simulink model "ShapeTracingSimExample"  (R2025b)
settings: Solver=VariableStepAuto  StartTime=0.0  StopTime=inf  RelTol=1e-3
InitFcn:
  | robotMesh = importrobot('ur5e_with_gripper.urdf');
undefined symbols (not defined in the file or in its folder): Sim3dSensor
libraries: sim3dlib x3, shareduavrstlib x1, sim3dphyssensorlib x1, robotsim3dlib x1, simulink x1, visionsinks x1
settings Model: Creator=The MathWorks, Inc.  LastModifiedBy=pepadev

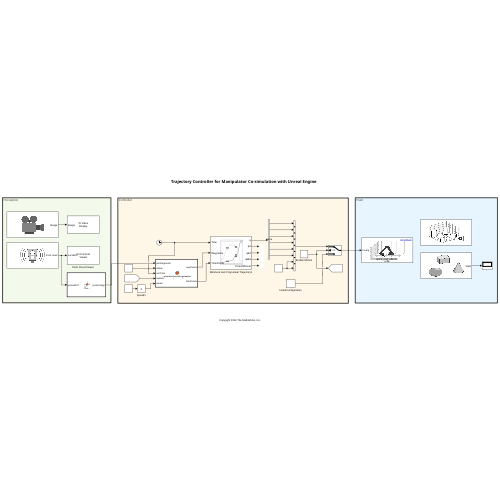
[thumbnail: Simulink's stored preview of the top-level diagram]
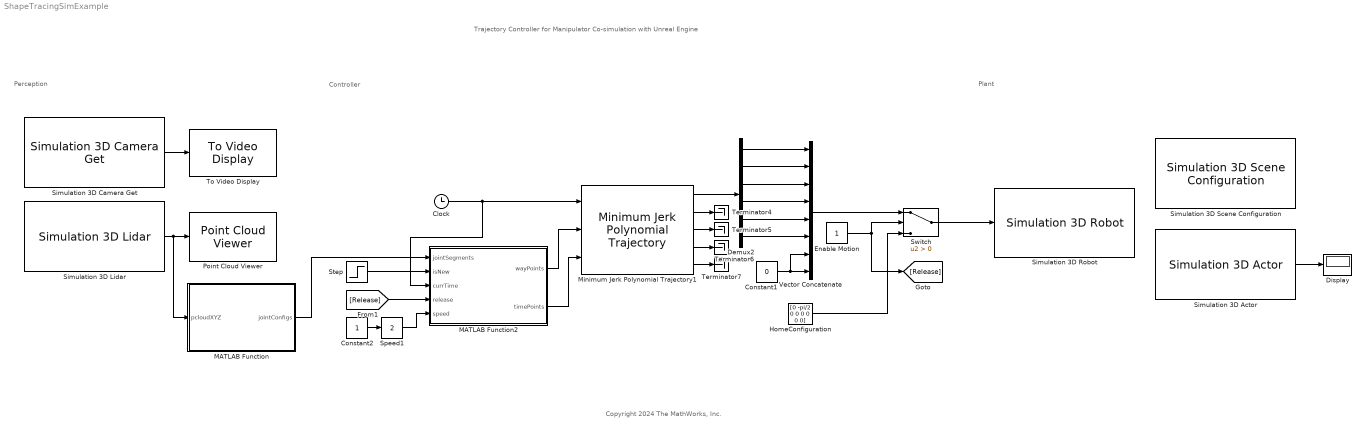
== system ShapeTracingSimExample ==
  note: Trajectory Controller for Manipulator Co-simulation with Unreal Engine
  note: Copyright 2024 The MathWorks, Inc.
  note: Plant
  note: Controller
  note: Perception
  Clock : Clock
  Constant1 : Constant  Value=0
  Constant2 : Constant
  Demux2 : Demux  Outputs=6
      settings: DisplayOption=none
  Display : Display
  Enable Motion : Constant
  HomeConfiguration : Constant  Value=|
      | [0
      | -pi/2
      | 0
      | 0
      | 0
      | 0
      | 0
      | 0]
  MATLAB Function : MATLAB Function  TreatAsAtomicUnit=on
  MATLAB Function2 : MATLAB Function  TreatAsAtomicUnit=on
  Minimum Jerk Polynomial Trajectory1 : shareduavrstlib/Minimum Jerk Polynomial Trajectory  ShowBCInputPort=off  ShowPolynomialCoefs=off  ShowStatusOutputPort=off  TimeAllocation=off  TimeWeight=100  MinSegmentTime=0.1  MaxSegmentTime=1  MaxIteration=1500  MaxTime=10  SimulateUsing=Interpreted execution
      settings: LibrarySourceBlock=robotutilslib/Minimum Jerk Polynomial Trajectory
  Point Cloud Viewer : PointCloudViewer  FigPos=[15.6666666666667 748.666666666667 1264 670.666666666667]  OpenAtMdlStart=off
  Simulation 3D Actor : sim3dlib/Simulation 3D Actor  Priority=1  ActorName=Actor1  ParentName=Scene Origin  Operation=Create at setup  InitScriptText=|  SampleTime=-1  Translation=single([0 0 0])  Rotation=single([0 0 0])  Scale=single([1 1 1])  aMode=5  ActorTag=Actor1  ActorType=Sim3dActor  ID=C
      | % Reserved keywords:
      | % - Actor : handle to this actor object
      | % - World : handle to the world object
      | 
      | % Examples:
      | 
      | % Create a primitive geometry (optional)
      | % Actor.createShape('box', [1 1 1]);
      | 
      | % Initialize values (optional)
      | % Actor.Scale = 1;
      | % Actor.Color = [1 0 0];
  Simulation 3D Camera Get : sim3dlib/Simulation 3D Camera Get  Priority=1  sensorTag=Sim3dSensor�  sensorId=1  sensorName=Sim3dSensor�  vehTagList={'Actor1';'Scene Origin';'ur5e'}  vehTag=ur5e  CoordinateSystem=Default  mountLoc=Origin  offsetFlag=on  tmountOffset=[- 5 0 3]  rmountOffset=[0 30 0]  HorizontalResolution=1280  VerticalResolution=720  HorizontalFOV=60  SampleTime=-1  mountPoint=[-5 0 3]  mountOrientation=[0 30 0]  aMode=5  ID=1
      settings: LibrarySourceBlock=sl3dlib/Simulation 3D/Utilities/Simulation 3D Camera Get
  Simulation 3D Lidar : sim3dphyssensorlib/Simulation 3D Lidar  Priority=1  sensorTag=Sim3dSensor�  sensorId=2  sensorName=Sim3dSensor�  vehTagList={'Actor1';'Scene Origin';'ur5e'}  vehTag=ur5e  CoordinateSystem=Default  mountLoc=Origin  offsetFlag=on  tmountOffset=[0, 0.25, 0.1]  rmountOffset=[0, 0, 90]  DetectionRange=1  RangeResolution=0.0001  VerticalFOV=48  VerticalResolution=0.1  HorizontalFOV=128  HorizontalResolution=0.2  DistanceOutportEnabled=off  ReflectivityOutportEnabled=off  SemanticOutportEnabled=off  TransformOutportEnabled=off  SampleTime=-1  mountPoint=[0 0.25 0.1]  mountOrientation=[0 0 90]  aMode=5  ID=2
      settings: LibrarySourceBlock=sl3dlib/Simulation 3D/Sensors/Simulation 3D Lidar
  Simulation 3D Robot : robotsim3dlib/Simulation 3D Robot  actorInputType=RigidBodyTree Object  RigidBodyTree=robotMesh  ActorName=ur5e  existActorChekBox=on  initialTrans=[ 4 2 0.55]  initialRot=[-pi/2 0 0]  initialConfig="[0  0  0  0  0  0  0  0]"  EndEffector=epick_end_effector  eeOffsetInpChekBox=off  eeTargetTrans=[0 0 0]  eeTargetRot=[0 0 0]  enableRegionGraspChekBox=off  regionGraspInpChekBox=off  eeTargTransDiff=[0.2 0.2 0.2]  eeTargRotDiff=[0 0 0]  enableVisualVisualization=on  enableCollisionVisualization=off  collisionGeomColor=[0 1 0]  collisionGeomTransp=0.1  inpConfEnbVal=on  inpGraspEnbVal=off  inpTransEnbVal=off  outConfEnbVal=off  outGraspEnbVal=off  outTransEnbVal=off  SampleTime=0.01  ActorType=SimulinkVehicle  ID=C  aMode=6  ActorTag=ur5e  Mesh=RigidBodyTree
  Simulation 3D Scene Configuration : sim3dlib/Simulation 3D Scene Configuration  Priority=0  ProjectFormat=Default Scenes  SceneDesc=Empty scene  ProjectName=/usr/local/MATLAB/R2025b/toolbox/shared/sim3d_projects/automotive_project_linux/UE/LinuxNoEditor/VehicleSimulation.sh  ScenePath=/Game/Maps/EmptyScene  EnableOpenDRIVE=off  vehTagList={'Actor1';'Custom';'Scene Origin';'ur5e'}  vehTag=Scene Origin  AttachedCameraRelativeTranslation=[0 0 0]  FreeCameraDefaultInitialTranslation=[-6, 0, 2]  AttachedCameraRelativeRotation=[0 0 0]  FreeCameraDefaultInitialRotation=[0, -15, 0]  ViewpointName=Custom  FreeCameraInitialTranslation=[0 -2 2]  ViewpointTranslation=[0 0 0]  FreeCameraInitialRotation=[0 0 0]  ViewpointRotation=[0 0 0]  OpVisEn=off  Ts=0.01  EnableWindow=on  EnableRemoteAccess=off  EnableWeather=off  SunAzimuth=90  SunAltitude=40.0  EnableGeospatialSun=off  Latitude=0  Longitude=0  Date=2023-01-01  Time=10:30:00  GeoTimeZone=-5.0  SunDaylightSaving=off  wind=1  clouds=10  EnableVolumetricClouds=off  CloudCoverage=0  CloudAltitude=6  fog=0  rain=0  RaindropsEffect=off  SnowDensity=0  EnableGeospatial=off  TilesetSource=Earth terrain  UseTrueOrigin=off  OriginHeight=200  OriginLatitude=40.744652  OriginLongitude=-73.988864  MapStyle=Aerial  AdditionalAssetIDs=[]  UseAdvancedSunSky=off  SolarTime=11  TimeZone=-5  Day=21  Month=9  Year=2022  UseDaylightSavingTime=on  DSTStartDay=10  DSTStartMonth=3  DSTEndDay=3  DSTEndMonth=11  DSTSwitchHour=2  sensorTag=MainCamera1  sensorId=1  sensorName=MainCamera1  mountLoc=Origin  offsetFlag=off  tmountOffset=[0, 0, 0]  rmountOffset=[0, 0, 0]  HorizontalResolution=1280  VerticalResolution=720  HorizontalFOV=60  mountPoint=[0 0 0]  mountOrientation=[0 0 0]  aMode=6  ID=1  GeoTrigger=Inactive  ViewNameList={'Custom'}  ViewTranslationList={'[0 -2 2]'}  ViewRotationList={'[0 0 0]'}
      settings: LibrarySourceBlock=robotsim3dlib/Simulation 3D Scene Configuration
  Speed1 : simulink/Math Operations/Slider Gain  gain=2  low=0  high=2
  Step : Step  Before=1  After=0  SampleTime=0.1
  Switch : Switch  Criteria=u2 > Threshold  SaturateOnIntegerOverflow=off  InputSameDT=off
  Terminator{4..7} (4 alike) : Terminator
  To Video Display : visionsinks/To Video Display  windowSizeMode=Normal  openAtMdlStart=on  fullScreen=off  videoWindowX=536805376  videoWindowY=536805376  saveWindowSize=off  videoWindowWidth=1280  videoWindowHeight=720  inputColorFormat=RGB  inputType=Obsolete  imagePorts=One multidimensional signal  OutputDevice=On-screen video monitor  dataOrg=Column-major  isWindowOpen=off
  Vector Concatenate : Concatenate  NumInputs=8
  wires:
  Simulation 3D Camera Get/1 -> To Video Display/1
  Simulation 3D Actor/1 -> Display/1
  Switch/1 -> Simulation 3D Robot/1
  Enable Motion/1 -> [Release], Switch/2
  HomeConfiguration/1 -> Switch/3
  Simulation 3D Lidar/1 -> MATLAB Function/1(pcloudXYZ), Point Cloud Viewer/1
  Vector Concatenate/1 -> Switch/1
  Constant1/1 -> Vector Concatenate/8, Vector Concatenate/7
  Clock/1 -> Minimum Jerk Polynomial Trajectory1/1, MATLAB Function2/3(currTime)
  Minimum Jerk Polynomial Trajectory1/1 -> Demux2/1
  MATLAB Function/1(jointConfigs) -> MATLAB Function2/1(jointSegments)
  Minimum Jerk Polynomial Trajectory1/4 -> Terminator6/1
  [Release] -> MATLAB Function2/4(release)
  Speed1/1 -> MATLAB Function2/5(speed)
  Minimum Jerk Polynomial Trajectory1/2 -> Terminator4/1
  MATLAB Function2/2(timePoints) -> Minimum Jerk Polynomial Trajectory1/3
  Step/1 -> MATLAB Function2/2(isNew)
  MATLAB Function2/1(wayPoints) -> Minimum Jerk Polynomial Trajectory1/2
  Minimum Jerk Polynomial Trajectory1/5 -> Terminator7/1
  Constant2/1 -> Speed1/1
  Minimum Jerk Polynomial Trajectory1/3 -> Terminator5/1
  Demux2/1 -> Vector Concatenate/1
  Demux2/2 -> Vector Concatenate/2
  Demux2/3 -> Vector Concatenate/3
  Demux2/4 -> Vector Concatenate/4
  Demux2/5 -> Vector Concatenate/5
  Demux2/6 -> Vector Concatenate/6

== matlab function ShapeTracingSimExample/MATLAB Function ==
  data: pcloudXYZ input; jointConfigs output double size=[6,120]
function jointConfigs  = fcn(pcloudXYZ)

jointConfigs = zeros([6,120]);

coder.extrinsic('evalin')
coder.extrinsic('helperGenerateJointConfig')
configExists = evalin('base','exist(''jointConfigs'',''var'')==1');

if ~configExists
    % Generate joint configuration only once based on scanned point cloud
    jointConfigs = helperGenerateJointConfig(pcloudXYZ);
else
    % Load joint configuration from MATLAB base workspace
    jointConfigs = evalin("base","jointConfigs");
end

end

== matlab function ShapeTracingSimExample/MATLAB Function2 ==
  data: jointSegments input; isNew input; wayPoints output; currTime input; release input; speed input; timePoints output
function [wayPoints,timePoints] = processJointSegments(jointSegments,isNew,currTime,release,speed)

persistent currStartTime idx currSegmentWayPoints currSegmentTimePoints dir sz
del = 0.5/speed;
if isempty(currStartTime)
    currStartTime = currTime;
    if isempty(currSegmentTimePoints)
        currSegmentTimePoints = linspace(currStartTime,currStartTime+del,2);
    end
end

if isempty(idx)
    idx = 1;
    if isempty(dir)
        dir = 2;
    end
    if isempty(currSegmentWayPoints)
        currSegmentWayPoints = jointSegments(:,[idx,idx+1]);
        sz = nnz(jointSegments)/6;
    end
end

if isNew
    idx = 1;
    dir = 2;
    sz = nnz(jointSegments)/6;
    currSegmentWayPoints = jointSegments(:,[idx,idx+1]);
end


if ~release 
    wayPoints = currSegmentWayPoints;
    timePoints = currSegmentTimePoints;
else
    if (currTime <= currStartTime+del)
        wayPoints = currSegmentWayPoints;
        timePoints = currSegmentTimePoints;
    else
        idx = idx + (-1)^dir;
        currStartTime = currTime;
        currSegmentTimePoints = linspace(currStartTime,currStartTime+del,2);
        currSegmentWayPoints = jointSegments(:,[idx,idx+(-1)^dir]);
        wayPoints = currSegmentWayPoints;
        timePoints = currSegmentTimePoints;
         if idx == sz-1 && dir == 2
            dir = 1;
            idx = idx + 1;
         elseif idx == 2 && dir == 1
             dir = 2;
         end
    end
end
end
